simulink model "model"  (R2019a)
settings: Solver=VariableStepAuto  StartTime=0.0  StopTime=20.0  RelTol=1e-3
libraries: mpclib x1, simulink x1
settings Model: Creator=alexh  LastModifiedBy=alexh
settings DebuggingCC: UnderSpecifiedDimensionMsg=warning

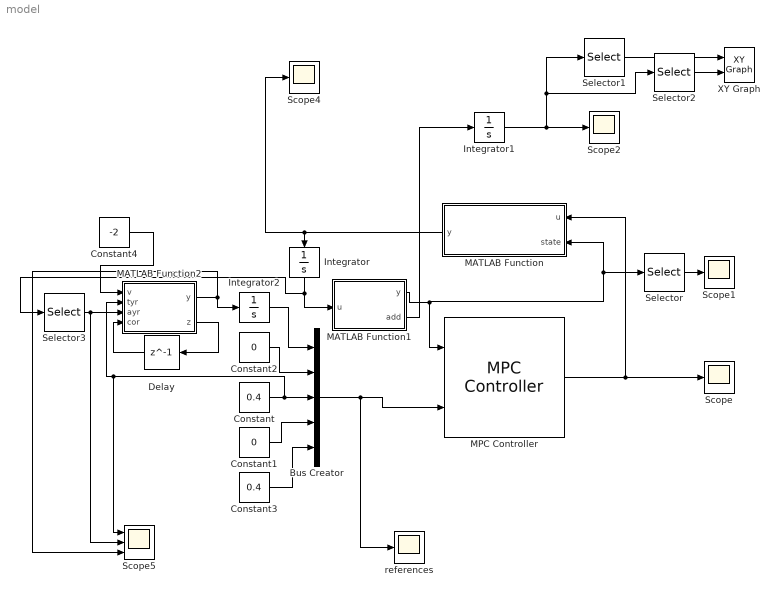
== system model ==
  Bus Creator : BusCreator  Inputs=5
  Constant : Constant  Value=0.4
  Constant1 : Constant  Value=0
  Constant2 : Constant  Value=0
  Constant3 : Constant  Value=0.4
  Constant4 : Constant  Value=-2
  Delay : Delay  DelayLength=1
  Integrator : Integrator
  Integrator1 : Integrator
  Integrator2 : Integrator  InitialCondition=-5
  MATLAB Function : MATLAB Function  TreatAsAtomicUnit=on
  MATLAB Function1 : MATLAB Function  TreatAsAtomicUnit=on
  MATLAB Function2 : MATLAB Function  TreatAsAtomicUnit=on
  MPC Controller : mpclib/MPC Controller  SCDEnableBlockLinearizationSpecification=on  mpcobj=mpc1  is_multiple=0  enable_value=0  return_u0=off  updateMPCinCallerWorkspace=on  md_inport=off  mv_inport=off  uref_inport=off  return_cost=off  return_mvseq=off  return_qpstatus=off  return_xseq=off  return_state=off  return_ovseq=off  state_inport=off  umin_inport=off  umax_inport=off  ymin_inport=off  ymax_inport=off  cc_inport=off  ywt_inport=off  uwt_inport=off  duwt_inport=off  rhoeps_inport=off  pm_inport=off  MaximumP=10  HorizonChoice=FixedHorizon  n_ts=0.1  n_p=10  n_mv=2  n_md=0  n_ud=0  n_mo=5  n_uo=0  BlockDataType=double  SampleTimeInherited=off  switch_inport=off
      settings: SourceProductName=MATLAB Runtime - Model Predictive Control Toolbox Addin  SourceProductBaseCode=Missing
  Scope{,1..2,4} (4 alike) : Scope
  Scope5 : Scope  NumInputPorts=3
  Selector : Selector  InputPortWidth=5  IndexOptions=Index vector (dialog)  Indices=[1 2 3 4]  OutputSizes=1
  Selector1 : Selector  InputPortWidth=3  IndexOptions=Index vector (dialog)  Indices=[1]  OutputSizes=1
  Selector2 : Selector  InputPortWidth=3  IndexOptions=Index vector (dialog)  Indices=[2]  OutputSizes=1
  Selector3 : Selector  InputPortWidth=5  IndexOptions=Index vector (dialog)  Indices=[3]  OutputSizes=1
  XY Graph : simulink/Sinks/XY Graph  xmin=-20  xmax=20  ymin=-20  ymax=20  st=-1
  references : Scope
  wires:
  Constant/1 -> Scope5/1, MATLAB Function2/2(tyr), Bus Creator/3
  Constant1/1 -> Bus Creator/4
  Bus Creator/1 -> references/1, MPC Controller/2
  MPC Controller/1 -> Scope/1, MATLAB Function/1(u)
  MATLAB Function/1(y) -> Scope4/1, Integrator/1
  Integrator/1 -> MATLAB Function1/1(u), Selector3/1
  Selector/1 -> Scope1/1
  Constant2/1 -> Bus Creator/2
  MATLAB Function1/1(y) -> Selector/1, MATLAB Function/2(state), MPC Controller/1
  Integrator1/1 -> Selector1/1, Selector2/1, Scope2/1
  Selector1/1 -> XY Graph/1
  Selector2/1 -> XY Graph/2
  MATLAB Function1/2(add) -> Integrator1/1
  Integrator2/1 -> Bus Creator/1
  Constant3/1 -> Bus Creator/5
  MATLAB Function2/2(z) -> Delay/1
  Constant4/1 -> MATLAB Function2/1(v)
  MATLAB Function2/1(y) -> Integrator2/1, Scope5/3
  Delay/1 -> MATLAB Function2/4(cor)
  Selector3/1 -> Scope5/2, MATLAB Function2/3(ayr)

== matlab function model/MATLAB Function1 ==
  data: u input; y output; add output
function [y, add]= fcn(u)

if u(1)>pi
    %u(1) = u(1) -2*pi;
end
if u(1)<-pi
    %u(1) = u(1) +2*pi;
end

y = u;

Vx = 2;
add = [cos(y(2))*Vx; sin(y(2))*Vx; y(3)];

== matlab function model/MATLAB Function ==
  data: u input; y output; state input
function y = fcn(u, state)

m = 30;     % Mass
lf = 0.7;   % Distance mass center/front wheel
lr = 0.3;   % Distance mass center/rear wheel
cf = 3000;   % Cornering Stiffness front
cr = 3000;   % Cornering Stiffness rear
iz = 100;   % Yaw Moment of Innertia

Vx = 2.0;

% Continuous-time model
Ac = [0, 0, Vx, 0, -Vx;
      0, 0, 1, 0, 0;
      0, 0, -(cr*lr^2+cf*lf^2)/(iz*Vx), -(cr*lr-cf*lf)/iz, 0;
      0, 0, 1-(cr*lr-cf*lf)/(m*Vx^2), -(cf+cr)/(m*Vx), 0;
      0, 0, 0, 0, -1];
   
Bc = [0, 0, cf*lf/iz, -cf/(m*Vx), 0;
      0, 0, 0, 0, -1]';

y = Ac*state + Bc*u;

== matlab function model/MATLAB Function2 ==
  data: v input; tyr input; ayr input; y output; cor input; z output
function [y, z]= fcn(v, tyr, ayr, cor)

correction_angle = (ayr-tyr);

y = correction_angle*v;
z = correction_angle;
